simulink model "system"  (R2024b)
settings: Solver=VariableStepAuto  StartTime=0.0  StopTime=20.0  RelTol=1e-3
values from neighbouring files (symbols this model uses):
  a = -H / (m * cp)    (= -0.00238891543239)    [Varmebad.m]    (also in variabler.m = -0.790959608031)
  b = P0 / (m * cp)    (= 0.11944577162)    [Varmebad.m]    (also in variabler.m = 0.074689292543)
  f = 50    [variabler.m]
  Kd = 0.05    [Varmebad.m]    (also in variabler.m = 1)
  Ki = 0.1    [Varmebad.m]    (also in variabler.m = 5)
  Kp = 2    [Varmebad.m]    (also in variabler.m = 5)
  P0 = 500    [Varmebad.m]    (also in variabler.m = 1500)
  T_0 = 23    [Varmebad.m]    (also in variabler.m = 20)
  T_a = 38    [Varmebad.m]    (also in variabler.m)
libraries: simulink x1
settings Model: Creator=ivers  LastModifiedBy=ivers

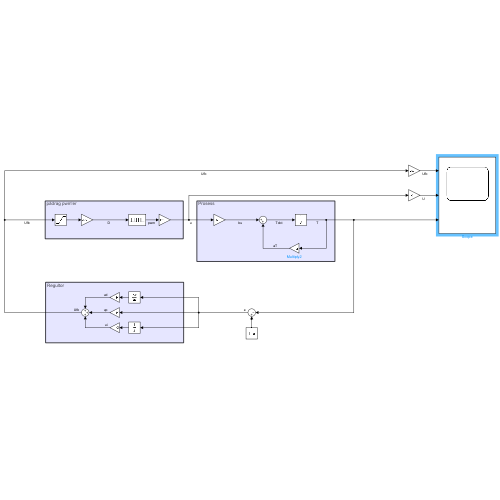
[thumbnail: Simulink's stored preview of the top-level diagram]
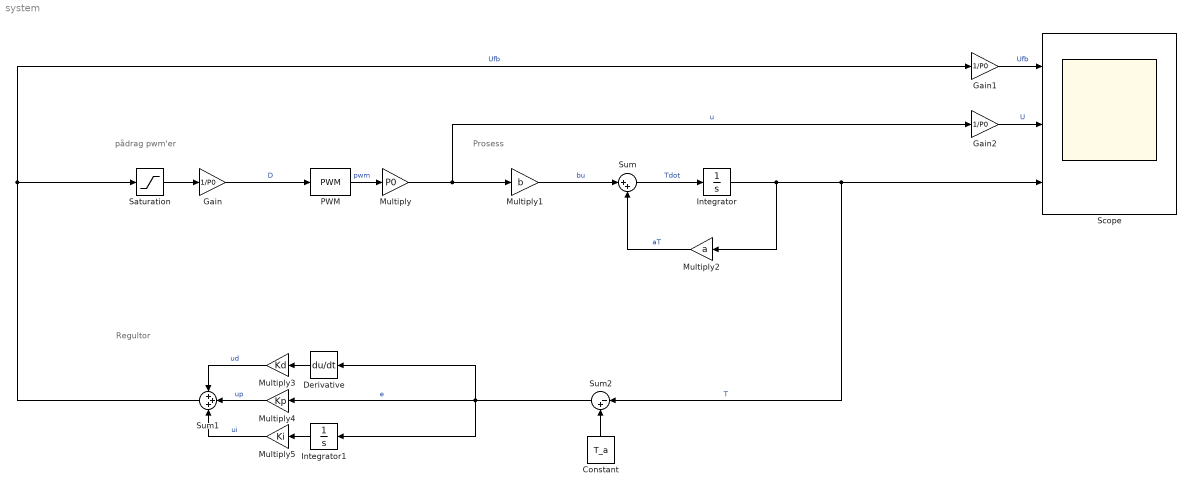
== system system ==
  note: Prosess
  note: pådrag pwm'er
  note: Regultor
  Constant : Constant  Value=T_a
  Derivative : Derivative
  Gain : Gain  Gain=1/P0
  Gain1 : Gain  Gain=1/P0
  Gain2 : Gain  Gain=1/P0
  Integrator : Integrator  InitialCondition=T_0
  Integrator1 : Integrator
  Multiply : Gain  Gain=P0
  Multiply1 : Gain  Gain=b
  Multiply2 : Gain  Gain=a
  Multiply3 : Gain  Gain=Kd
  Multiply4 : Gain  Gain=Kp
  Multiply5 : Gain  Gain=Ki
  PWM : simulink/Discontinuities/PWM  DisableCoverage=on  Period=1/f  InitialDelay=0  DisallowZeroDutyCycle=off  RunAtFixedTimeIntervals=off  SampleTime=0.1
  Saturation : Saturate  UpperLimit=P0  LowerLimit=0
  Scope : Scope  NumInputPorts=3
  Sum : Sum  Inputs=|++
  Sum1 : Sum  Inputs=+++
  Sum2 : Sum  Inputs=|-+
  wires:
  Saturation/1 -> Gain/1
  Gain/1 -> PWM/1  "D"
  PWM/1 -> Multiply/1  "pwm"
  Multiply/1 -> Gain2/1, Multiply1/1  "u"
  Multiply1/1 -> Sum/1  "bu"
  Sum/1 -> Integrator/1  "Tdot"
  Integrator/1 -> Multiply2/1, Sum2/1, Scope/3  "T"
  Multiply2/1 -> Sum/2  "aT"
  Integrator1/1 -> Multiply5/1
  Multiply3/1 -> Sum1/1  "ud"
  Multiply4/1 -> Sum1/2  "up"
  Multiply5/1 -> Sum1/3  "ui"
  Sum1/1 -> Gain1/1, Saturation/1  "Ufb"
  Sum2/1 -> Integrator1/1, Multiply4/1, Derivative/1  "e"
  Derivative/1 -> Multiply3/1
  Constant/1 -> Sum2/2
  Gain1/1 -> Scope/1  "Ufb"
  Gain2/1 -> Scope/2  "U"
